simulink library "lookUpTable"  (R2016b)
settings: Solver=VariableStepAuto  StartTime=0.0  StopTime=10.0  RelTol=1e-3
undefined symbols (not defined in the file or in its folder): halfStepStandStartHip, halfStepStandStartKnee, halfStepStopFromStandHip, halfStepStopFromStandKnee, halfStepStopFromSwingHip, halfStepStopFromSwingKnee, halfStepSwingStartHip, halfStepSwingStartKnee, sitDownHip, sitDownKnee, standUpHip, standUpKnee, stepStandLegHip, stepStandLegKnee, stepSwingLegHip, stepSwingLegKnee
libraries: lookUpTotalGaitDynamics x5
settings Model: Creator=Nathan  LastModifiedBy=Taeke

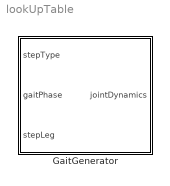
== system lookUpTable ==
  GaitGenerator : Subsystem

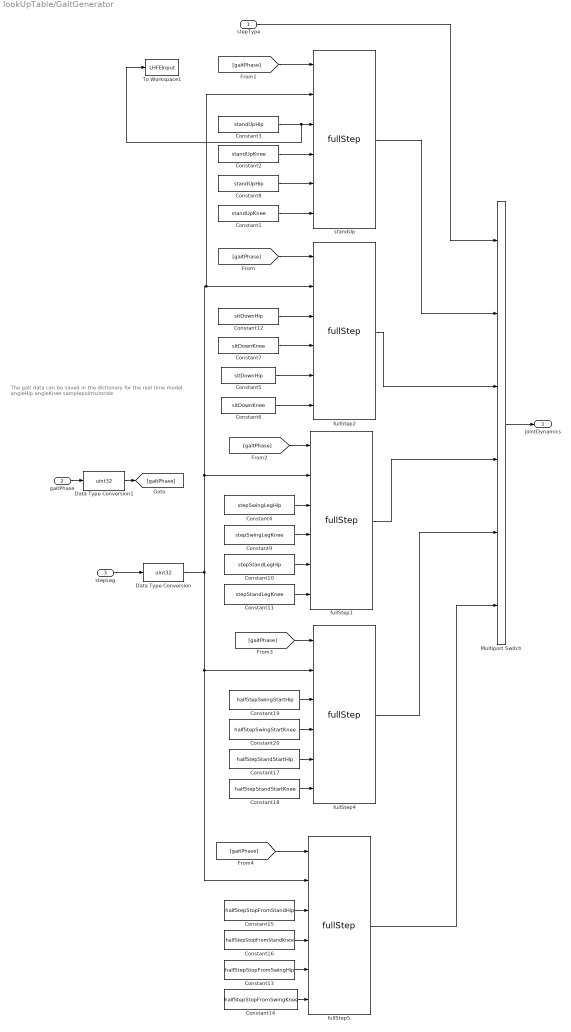
== system lookUpTable/GaitGenerator ==
  note: The gait data can be saved in the dictionary for the real time model
      | angleHip
      | angleKnee
      | samplepoints/stride
  stepType : Inport
  gaitPhase : Inport  Port=2
  stepLeg : Inport  Port=3
  Constant1 : Constant  Value=standUpKnee
  Constant10 : Constant  Value=stepStandLegHip
  Constant11 : Constant  Value=stepStandLegKnee
  Constant12 : Constant  Value=sitDownHip
  Constant13 : Constant  Value=halfStepStopFromSwingHip
  Constant14 : Constant  Value=halfStepStopFromSwingKnee
  Constant15 : Constant  Value=halfStepStopFromStandHip
  Constant16 : Constant  Value=halfStepStopFromStandKnee
  Constant17 : Constant  Value=halfStepStandStartHip
  Constant18 : Constant  Value=halfStepStandStartKnee
  Constant19 : Constant  Value=halfStepSwingStartHip
  Constant2 : Constant  Value=standUpKnee
  Constant20 : Constant  Value=halfStepSwingStartKnee
  Constant3 : Constant  Value=standUpHip
  Constant4 : Constant  Value=stepSwingLegHip
  Constant5 : Constant  Value=sitDownHip
  Constant6 : Constant  Value=sitDownKnee
  Constant7 : Constant  Value=sitDownKnee
  Constant8 : Constant  Value=standUpHip
  Constant9 : Constant  Value=stepSwingLegKnee
  Data Type Conversion : DataTypeConversion  OutDataTypeStr=uint32
  Data Type Conversion1 : DataTypeConversion  OutDataTypeStr=uint32  RndMeth=Nearest
  Multiport Switch : MultiPortSwitch  DataPortOrder=Specify indices  Inputs=4  DataPortIndices={StepType.STANDUP,StepType.SITDOWN,StepType.FULLSTEP,StepType.HALFSTEPSTART,StepType.HALFSTEPSTOP,}  DiagnosticForDefault=None
  To Workspace1 : ToWorkspace  VariableName=LHFEInput  SaveFormat=Timeseries  SampleTime=-1
  fullStep{1..2,4..5} (4 alike) : lookUpTotalGaitDynamics/fullStep
  standUp : lookUpTotalGaitDynamics/fullStep
  jointDynamics : Outport  OutDataTypeStr=Bus: JointDynamics
  wires:
  gaitPhase/1 -> Data Type Conversion1/1
  Constant3/1 -> standUp/3, To Workspace1/1
  Data Type Conversion1/1 -> [gaitPhase]
  [gaitPhase] -> fullStep5/1
  Constant14/1 -> fullStep5/6
  Constant13/1 -> fullStep5/5
  Constant16/1 -> fullStep5/4
  Constant15/1 -> fullStep5/3
  Constant18/1 -> fullStep4/6
  Constant17/1 -> fullStep4/5
  Constant20/1 -> fullStep4/4
  Constant19/1 -> fullStep4/3
  Data Type Conversion/1 -> fullStep4/2, fullStep5/2, fullStep2/2, standUp/2, fullStep1/2
  Constant12/1 -> fullStep2/3
  Constant7/1 -> fullStep2/4
  Constant2/1 -> standUp/4
  Constant8/1 -> standUp/5
  Constant1/1 -> standUp/6
  Constant11/1 -> fullStep1/6
  [gaitPhase] -> fullStep4/1
  [gaitPhase] -> fullStep1/1
  [gaitPhase] -> standUp/1
  [gaitPhase] -> fullStep2/1
  Constant6/1 -> fullStep2/6
  Constant5/1 -> fullStep2/5
  Constant10/1 -> fullStep1/5
  Constant9/1 -> fullStep1/4
  Constant4/1 -> fullStep1/3
  fullStep5/1 -> Multiport Switch/6
  fullStep4/1 -> Multiport Switch/5
  fullStep1/1 -> Multiport Switch/4
  Multiport Switch/1 -> jointDynamics/1
  standUp/1 -> Multiport Switch/2
  stepType/1 -> Multiport Switch/1
  fullStep2/1 -> Multiport Switch/3
  stepLeg/1 -> Data Type Conversion/1
